simulink model "LABORATORY2"  (R2024b)
settings: Solver=VariableStepAuto  StartTime=0.0  StopTime=10.0  RelTol=1e-3
undefined symbols (not defined in the file): b1, b2, k1, k2, M1, M2
settings Model: Creator=Admin  LastModifiedBy=Admin

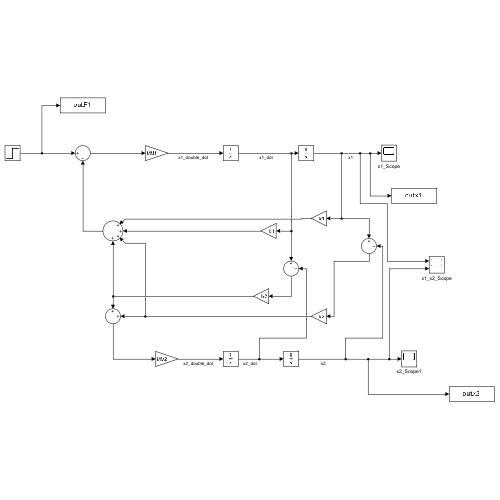
[thumbnail: Simulink's stored preview of the top-level diagram]
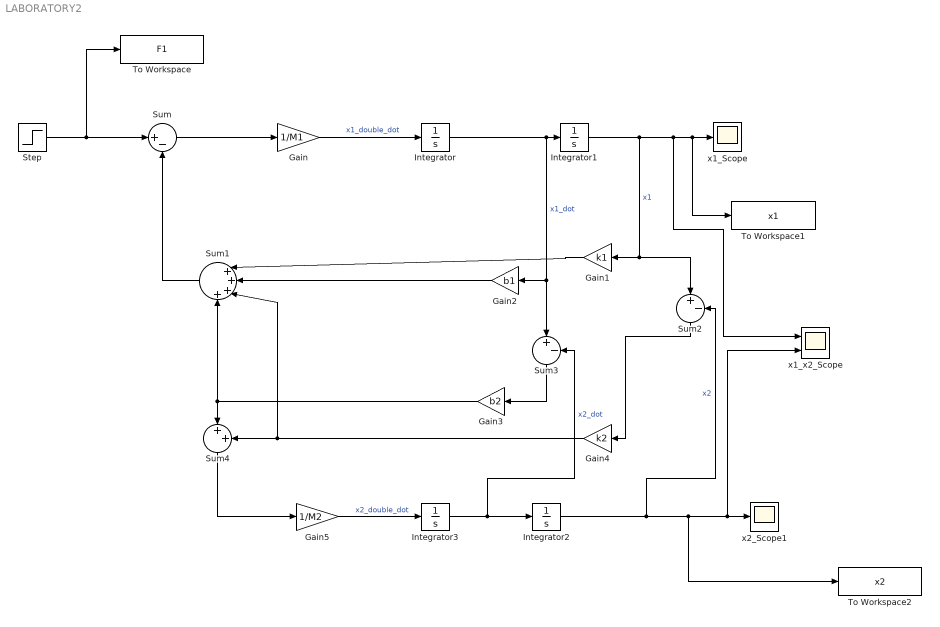
== system LABORATORY2 ==
  Gain : Gain  Gain=1/M1
  Gain1 : Gain  Gain=k1
  Gain2 : Gain  Gain=b1
  Gain3 : Gain  Gain=b2
  Gain4 : Gain  Gain=k2
  Gain5 : Gain  Gain=1/M2
  Integrator{,1..3} (4 alike) : Integrator
  Step : Step  SampleTime=0
  Sum : Sum  Inputs=|+-
  Sum1 : Sum  Inputs=|++++
  Sum2 : Sum  Inputs=|+-
  Sum3 : Sum  Inputs=|+-
  Sum4 : Sum  Inputs=|++
  To Workspace : ToWorkspace  VariableName=F1  SaveFormat=Timeseries  SampleTime=-1
  To Workspace1 : ToWorkspace  VariableName=x1  SaveFormat=Timeseries  SampleTime=-1
  To Workspace2 : ToWorkspace  VariableName=x2  SaveFormat=Timeseries  SampleTime=-1
  x1_Scope : Scope
  x1_x2_Scope : Scope  NumInputPorts=2
  x2_Scope1 : Scope
  wires:
  Step/1 -> To Workspace/1, Sum/1
  Sum/1 -> Gain/1
  Gain/1 -> Integrator/1  "x1_double_dot"
  Integrator/1 -> Integrator1/1, Sum3/1, Gain2/1  "x1_dot"
  Integrator1/1 -> x1_x2_Scope/1, x1_Scope/1, To Workspace1/1, Sum2/1, Gain1/1  "x1"
  Sum1/1 -> Sum/2
  Gain1/1 -> Sum1/1
  Gain2/1 -> Sum1/2
  Sum3/1 -> Gain3/1
  Gain3/1 -> Sum4/1, Sum1/4
  Gain4/1 -> Sum4/2, Sum1/3
  Sum2/1 -> Gain4/1
  Integrator2/1 -> Sum2/2, To Workspace2/1, x1_x2_Scope/2, x2_Scope1/1  "x2"
  Sum4/1 -> Gain5/1
  Gain5/1 -> Integrator3/1  "x2_double_dot"
  Integrator3/1 -> Sum3/2, Integrator2/1  "x2_dot"
